simulink model "ejemplo_simulink"  (R2018b)
settings: Solver=VariableStepAuto  StartTime=0.0  StopTime=10.0  RelTol=1e-3
settings Model: Creator=carta  LastModifiedBy=carta

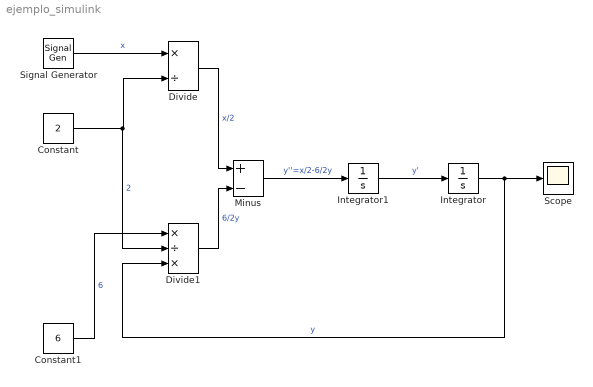
== system ejemplo_simulink ==
  Constant : Constant  Value=2
  Constant1 : Constant  Value=6
  Divide : Product  Inputs=*/
  Divide1 : Product  Inputs=*/*
  Integrator : Integrator
  Integrator1 : Integrator
  Minus : Sum  Inputs=+-
  Scope : Scope
  Signal Generator : SignalGenerator  WaveForm=square  Units=rad/sec
  wires:
  Integrator/1 -> Divide1/3, Scope/1  "y"
  Integrator1/1 -> Integrator/1  "y'"
  Minus/1 -> Integrator1/1  "y''=x/2-6/2y"
  Signal Generator/1 -> Divide/1  "x"
  Constant/1 -> Divide1/2, Divide/2  "2"
  Divide/1 -> Minus/1  "x/2"
  Constant1/1 -> Divide1/1  "6"
  Divide1/1 -> Minus/2  "6/2y"
